simulink model "IEEE34_SPSload"  (R2021b)
settings: Solver=ode4  StartTime=0.0  StopTime=5  FixedStep=50e-6  RelTol=1e-3
PreLoadFcn:
  | pGain = 0.05; % Gain of random perturbation (pu)
  | pGainAP = 0.01; % Gain of sinusoidal active power variation (pu)
  | pGainRP = 0.01; % Gain of sinusoidal reactive power variation (pu)
  | pFreqAP = 0.03; % Frequency of sinusoidal active power variation (Hz)
  | pFreqRP = 0.03; % Frequency of sinusoidal reactive power variation (Hz)
  | 
  | init_IEEE34nodetestfeeder;
InitFcn:
  | pGain = 0.05; % Gain of random perturbation (pu)
  | pGainAP = 0.01; % Gain of sinusoidal active power variation (pu)
  | pGainRP = 0.01; % Gain of sinusoidal reactive power variation (pu)
  | pFreqAP = 0.03; % Frequency of sinusoidal active power variation (Hz)
  | pFreqRP = 0.03; % Frequency of sinusoidal reactive power variation (Hz)
  | 
  | init_IEEE34nodetestfeeder;
values from neighbouring files (symbols this model uses):
  fNom = f    (= 60)    [init_IEEE34nodetestfeeder.m]
  loadcoeff = 1.0    (= 1)    [init_IEEE34nodetestfeeder.m]
  Ts = 50e-6    (= 5e-05)    [init_IEEE34nodetestfeeder.m]
  vNomMV = VsubL    (= 24900)    [init_IEEE34nodetestfeeder.m]
  VsubL = 24.9e3    (= 24900)    [init_IEEE34nodetestfeeder.m]
  VxfmL = 4.16e3    (= 4160)    [init_IEEE34nodetestfeeder.m]
undefined symbols (not defined in the file or in its folder): Ac, Bc, Cc, Dc, find_system, j
libraries: spsSeriesRLCBranchLib x418, spsGroundLib x242, simulink_extras x176, spsVoltageMeasurementLib x106, spsRMSLib x96, spsControlledCurrentSourceLib x94, spsThreePhaseVIMeasurementLib x37, spsMutualInductanceLib x24, spsCurrentMeasurementLib x12, spsOnDelayLib x12, spsLinearTransformerLib x6, spsControlledVoltageSourceLib x6
(part 8 of 33)

== system IEEE34_SPSload/SM_IEEE34/Spot 830 ==
  Load B : Subsystem  DialogController=POWERSYS.PowerSysDialog  mask(Single-Phase Dynamic Load){NominalVoltage=[ VsubL 60 ], ActiveReactivePowers=[10*1000*loadcoeff 5*1000*loadcoeff], PositiveSequence=[1 0], ExternalControl=off, NpNq=[2 2], TimeConstants=[0  0  0  0], MinimumVoltage=0.7, LoadFlowParameters=[4,0,0,0,0]}
      mask prompts: NominalVoltage "Nominal voltage and frequency  [Vn(Vrms) fn(Hz)]:"; ActiveReactivePowers "Active and reactive power at initial voltage [Po(W) Qo(var)]:"; PositiveSequence "Initial voltage Vo [Mag(pu) Phase (deg.)]:"; ExternalControl "External control of PQ"; NpNq "Parameters [ np  nq ]:"; TimeConstants "Time constants [Tp1 Tp2 Tq1 Tq2]  (s):"; MinimumVoltage "Minimum voltage Vmin (pu):"; LoadFlowParameters "Load Flow parameters"
      mask help:
      | Implements a single-phase dynamic load. Active  power P and reactive
      | power Q absorbed by the load vary as function of voltage V  according to the
      | following equations:
      |
      |   If V>Vmin, P and Q vary as follows:
      |        P = Po * (V/Vo)^np * (1+Tp1.s)/(1+Tp2.s)
      |        Q = Qo * (V/Vo)^nq * (1+Tq1.s)/(1+Tq2.s)
      |   if V<Vmin
      |      Same equations with np=nq=2 (constant impedance load)
      mask init: same as IEEE34_SPSload/SM_IEEE34/DL836-1/Load B
      mask Help: helpview(psbhelp)
      mask Callback ExternalControl: powericon('ThreePhaseDynamicLoadCback',gcb);
      mask Display:
      | plot(-45,-45,45,45,[0,9,18,24,29,30,29,24,18,9,0,-9,-18,-24,-29,-30,-29,-24,-18,-9,0]*.9,[30,29,24,18,9,0,-9,-18,-24,-29,-30,-29,-24,-18,-9,0,9,18,24,29,30]*.9)
      | plot([0,0,10,0,-10,0]*1.1,[15,-5,-5,-15,-5,-5]*1.1)
  Load B1 : Subsystem  DialogController=POWERSYS.PowerSysDialog  mask(Single-Phase Dynamic Load){NominalVoltage=[ VsubL 60 ], ActiveReactivePowers=[10*1000*loadcoeff 5*1000*loadcoeff], PositiveSequence=[1 0], ExternalControl=off, NpNq=[2 2], TimeConstants=[0  0  0  0], MinimumVoltage=0.7, LoadFlowParameters=[4,0,0,0,0]}
      mask prompts: NominalVoltage "Nominal voltage and frequency  [Vn(Vrms) fn(Hz)]:"; ActiveReactivePowers "Active and reactive power at initial voltage [Po(W) Qo(var)]:"; PositiveSequence "Initial voltage Vo [Mag(pu) Phase (deg.)]:"; ExternalControl "External control of PQ"; NpNq "Parameters [ np  nq ]:"; TimeConstants "Time constants [Tp1 Tp2 Tq1 Tq2]  (s):"; MinimumVoltage "Minimum voltage Vmin (pu):"; LoadFlowParameters "Load Flow parameters"
      mask help:
      | Implements a single-phase dynamic load. Active  power P and reactive
      | power Q absorbed by the load vary as function of voltage V  according to the
      | following equations:
      |
      |   If V>Vmin, P and Q vary as follows:
      |        P = Po * (V/Vo)^np * (1+Tp1.s)/(1+Tp2.s)
      |        Q = Qo * (V/Vo)^nq * (1+Tq1.s)/(1+Tq2.s)
      |   if V<Vmin
      |      Same equations with np=nq=2 (constant impedance load)
      mask init: same as IEEE34_SPSload/SM_IEEE34/DL836-1/Load B
      mask Help: helpview(psbhelp)
      mask Callback ExternalControl: powericon('ThreePhaseDynamicLoadCback',gcb);
      mask Display:
      | plot(-45,-45,45,45,[0,9,18,24,29,30,29,24,18,9,0,-9,-18,-24,-29,-30,-29,-24,-18,-9,0]*.9,[30,29,24,18,9,0,-9,-18,-24,-29,-30,-29,-24,-18,-9,0,9,18,24,29,30]*.9)
      | plot([0,0,10,0,-10,0]*1.1,[15,-5,-5,-15,-5,-5]*1.1)
  Load B2 : Subsystem  DialogController=POWERSYS.PowerSysDialog  mask(Single-Phase Dynamic Load){NominalVoltage=[ VsubL 60 ], ActiveReactivePowers=[25*1000*loadcoeff 10*1000*loadcoeff], PositiveSequence=[1 0], ExternalControl=off, NpNq=[2 2], TimeConstants=[0  0  0  0], MinimumVoltage=0.7, LoadFlowParameters=[4,0,0,0,0]}
      mask prompts: NominalVoltage "Nominal voltage and frequency  [Vn(Vrms) fn(Hz)]:"; ActiveReactivePowers "Active and reactive power at initial voltage [Po(W) Qo(var)]:"; PositiveSequence "Initial voltage Vo [Mag(pu) Phase (deg.)]:"; ExternalControl "External control of PQ"; NpNq "Parameters [ np  nq ]:"; TimeConstants "Time constants [Tp1 Tp2 Tq1 Tq2]  (s):"; MinimumVoltage "Minimum voltage Vmin (pu):"; LoadFlowParameters "Load Flow parameters"
      mask help:
      | Implements a single-phase dynamic load. Active  power P and reactive
      | power Q absorbed by the load vary as function of voltage V  according to the
      | following equations:
      |
      |   If V>Vmin, P and Q vary as follows:
      |        P = Po * (V/Vo)^np * (1+Tp1.s)/(1+Tp2.s)
      |        Q = Qo * (V/Vo)^nq * (1+Tq1.s)/(1+Tq2.s)
      |   if V<Vmin
      |      Same equations with np=nq=2 (constant impedance load)
      mask init: same as IEEE34_SPSload/SM_IEEE34/DL836-1/Load B
      mask Help: helpview(psbhelp)
      mask Callback ExternalControl: powericon('ThreePhaseDynamicLoadCback',gcb);
      mask Display:
      | plot(-45,-45,45,45,[0,9,18,24,29,30,29,24,18,9,0,-9,-18,-24,-29,-30,-29,-24,-18,-9,0]*.9,[30,29,24,18,9,0,-9,-18,-24,-29,-30,-29,-24,-18,-9,0,9,18,24,29,30]*.9)
      | plot([0,0,10,0,-10,0]*1.1,[15,-5,-5,-15,-5,-5]*1.1)
  Terminator : Terminator
  Terminator1 : Terminator
  Terminator2 : Terminator
  A : PMIOPort  Side=Right
  B : PMIOPort  Port=2  Side=Right
  C : PMIOPort  Port=3  Side=Right
  wires:
  Load B/1(m) -> Terminator/1
  Load B1/1(m) -> Terminator1/1
  Load B2/1(m) -> Terminator2/1
  connections:
  A/RConn1 -- Load B2/LConn2 -- Load B/LConn1
  B/RConn1 -- Load B/LConn2 -- Load B1/LConn1
  C/RConn1 -- Load B1/LConn2 -- Load B2/LConn1

== system IEEE34_SPSload/SM_IEEE34/Spot 840 ==
  Ground4 : spsGroundLib/Ground  LConnTagsString=a
  Ground5 : spsGroundLib/Ground  LConnTagsString=a
  Ground6 : spsGroundLib/Ground  LConnTagsString=a
  Load B : Subsystem  DialogController=POWERSYS.PowerSysDialog  mask(Single-Phase Dynamic Load){NominalVoltage=[ VsubL/sqrt(3) 60 ], ActiveReactivePowers=[9*1000*loadcoeff 7*1000*loadcoeff], PositiveSequence=[1 0], ExternalControl=off, NpNq=[1 1], TimeConstants=[0  0  0  0], MinimumVoltage=0.7, LoadFlowParameters=[4,0,0,0,0]}
      mask prompts: NominalVoltage "Nominal voltage and frequency  [Vn(Vrms) fn(Hz)]:"; ActiveReactivePowers "Active and reactive power at initial voltage [Po(W) Qo(var)]:"; PositiveSequence "Initial voltage Vo [Mag(pu) Phase (deg.)]:"; ExternalControl "External control of PQ"; NpNq "Parameters [ np  nq ]:"; TimeConstants "Time constants [Tp1 Tp2 Tq1 Tq2]  (s):"; MinimumVoltage "Minimum voltage Vmin (pu):"; LoadFlowParameters "Load Flow parameters"
      mask help:
      | Implements a single-phase dynamic load. Active  power P and reactive
      | power Q absorbed by the load vary as function of voltage V  according to the
      | following equations:
      |
      |   If V>Vmin, P and Q vary as follows:
      |        P = Po * (V/Vo)^np * (1+Tp1.s)/(1+Tp2.s)
      |        Q = Qo * (V/Vo)^nq * (1+Tq1.s)/(1+Tq2.s)
      |   if V<Vmin
      |      Same equations with np=nq=2 (constant impedance load)
      mask init: same as IEEE34_SPSload/SM_IEEE34/DL836-1/Load B
      mask Help: helpview(psbhelp)
      mask Callback ExternalControl: powericon('ThreePhaseDynamicLoadCback',gcb);
      mask Display:
      | plot(-45,-45,45,45,[0,9,18,24,29,30,29,24,18,9,0,-9,-18,-24,-29,-30,-29,-24,-18,-9,0]*.9,[30,29,24,18,9,0,-9,-18,-24,-29,-30,-29,-24,-18,-9,0,9,18,24,29,30]*.9)
      | plot([0,0,10,0,-10,0]*1.1,[15,-5,-5,-15,-5,-5]*1.1)
  Load B1 : Subsystem  DialogController=POWERSYS.PowerSysDialog  mask(Single-Phase Dynamic Load){NominalVoltage=[ VsubL/sqrt(3) 60 ], ActiveReactivePowers=[9*1000*loadcoeff 7*1000*loadcoeff], PositiveSequence=[1 0], ExternalControl=off, NpNq=[1 1], TimeConstants=[0  0  0  0], MinimumVoltage=0.7, LoadFlowParameters=[4,0,0,0,0]}
      mask prompts: NominalVoltage "Nominal voltage and frequency  [Vn(Vrms) fn(Hz)]:"; ActiveReactivePowers "Active and reactive power at initial voltage [Po(W) Qo(var)]:"; PositiveSequence "Initial voltage Vo [Mag(pu) Phase (deg.)]:"; ExternalControl "External control of PQ"; NpNq "Parameters [ np  nq ]:"; TimeConstants "Time constants [Tp1 Tp2 Tq1 Tq2]  (s):"; MinimumVoltage "Minimum voltage Vmin (pu):"; LoadFlowParameters "Load Flow parameters"
      mask help:
      | Implements a single-phase dynamic load. Active  power P and reactive
      | power Q absorbed by the load vary as function of voltage V  according to the
      | following equations:
      |
      |   If V>Vmin, P and Q vary as follows:
      |        P = Po * (V/Vo)^np * (1+Tp1.s)/(1+Tp2.s)
      |        Q = Qo * (V/Vo)^nq * (1+Tq1.s)/(1+Tq2.s)
      |   if V<Vmin
      |      Same equations with np=nq=2 (constant impedance load)
      mask init: same as IEEE34_SPSload/SM_IEEE34/DL836-1/Load B
      mask Help: helpview(psbhelp)
      mask Callback ExternalControl: powericon('ThreePhaseDynamicLoadCback',gcb);
      mask Display:
      | plot(-45,-45,45,45,[0,9,18,24,29,30,29,24,18,9,0,-9,-18,-24,-29,-30,-29,-24,-18,-9,0]*.9,[30,29,24,18,9,0,-9,-18,-24,-29,-30,-29,-24,-18,-9,0,9,18,24,29,30]*.9)
      | plot([0,0,10,0,-10,0]*1.1,[15,-5,-5,-15,-5,-5]*1.1)
  Load B2 : Subsystem  DialogController=POWERSYS.PowerSysDialog  mask(Single-Phase Dynamic Load){NominalVoltage=[ VsubL/sqrt(3) 60 ], ActiveReactivePowers=[9*1000*loadcoeff 7*1000*loadcoeff], PositiveSequence=[1 0], ExternalControl=off, NpNq=[1 1], TimeConstants=[0  0  0  0], MinimumVoltage=0.7, LoadFlowParameters=[4,0,0,0,0]}
      mask prompts: NominalVoltage "Nominal voltage and frequency  [Vn(Vrms) fn(Hz)]:"; ActiveReactivePowers "Active and reactive power at initial voltage [Po(W) Qo(var)]:"; PositiveSequence "Initial voltage Vo [Mag(pu) Phase (deg.)]:"; ExternalControl "External control of PQ"; NpNq "Parameters [ np  nq ]:"; TimeConstants "Time constants [Tp1 Tp2 Tq1 Tq2]  (s):"; MinimumVoltage "Minimum voltage Vmin (pu):"; LoadFlowParameters "Load Flow parameters"
      mask help:
      | Implements a single-phase dynamic load. Active  power P and reactive
      | power Q absorbed by the load vary as function of voltage V  according to the
      | following equations:
      |
      |   If V>Vmin, P and Q vary as follows:
      |        P = Po * (V/Vo)^np * (1+Tp1.s)/(1+Tp2.s)
      |        Q = Qo * (V/Vo)^nq * (1+Tq1.s)/(1+Tq2.s)
      |   if V<Vmin
      |      Same equations with np=nq=2 (constant impedance load)
      mask init: same as IEEE34_SPSload/SM_IEEE34/DL836-1/Load B
      mask Help: helpview(psbhelp)
      mask Callback ExternalControl: powericon('ThreePhaseDynamicLoadCback',gcb);
      mask Display:
      | plot(-45,-45,45,45,[0,9,18,24,29,30,29,24,18,9,0,-9,-18,-24,-29,-30,-29,-24,-18,-9,0]*.9,[30,29,24,18,9,0,-9,-18,-24,-29,-30,-29,-24,-18,-9,0,9,18,24,29,30]*.9)
      | plot([0,0,10,0,-10,0]*1.1,[15,-5,-5,-15,-5,-5]*1.1)
  Terminator : Terminator
  Terminator1 : Terminator
  Terminator2 : Terminator
  A : PMIOPort  Side=Right
  B : PMIOPort  Port=2  Side=Right
  C : PMIOPort  Port=3  Side=Right
  wires:
  Load B/1(m) -> Terminator/1
  Load B1/1(m) -> Terminator1/1
  Load B2/1(m) -> Terminator2/1
  connections:
  Load B/LConn2 -- Ground4/LConn1
  A/RConn1 -- Load B/LConn1
  Load B1/LConn2 -- Ground5/LConn1
  B/RConn1 -- Load B1/LConn1
  C/RConn1 -- Load B2/LConn1
  Load B2/LConn2 -- Ground6/LConn1

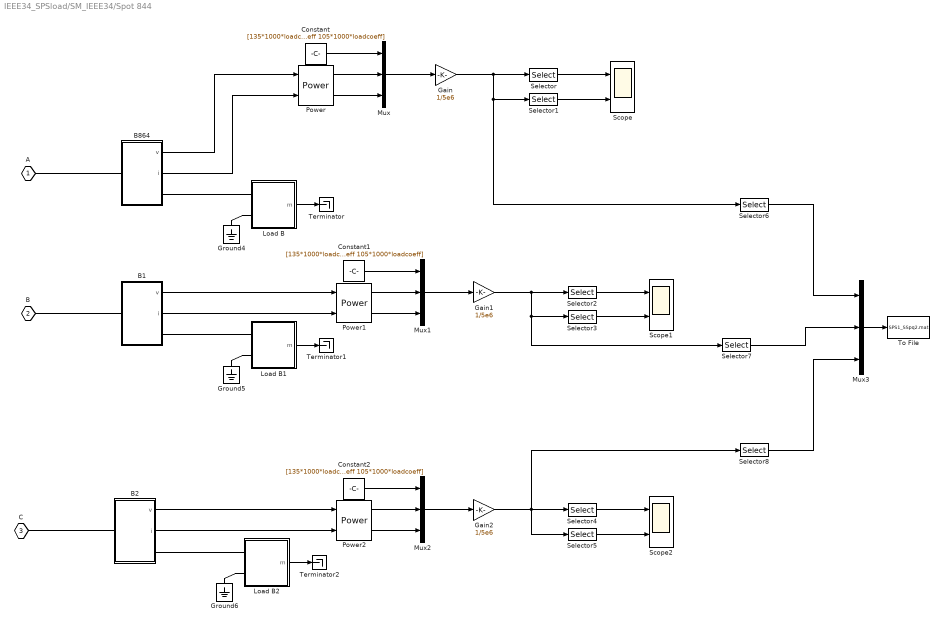
== system IEEE34_SPSload/SM_IEEE34/Spot 844 ==
  B1 : Subsystem
  B2 : Subsystem
  B864 : Subsystem
  Constant : Constant  Value=[135*1000*loadcoeff 105*1000*loadcoeff]
  Constant1 : Constant  Value=[135*1000*loadcoeff 105*1000*loadcoeff]
  Constant2 : Constant  Value=[135*1000*loadcoeff 105*1000*loadcoeff]
  Gain : Gain  Gain=1/5e6
  Gain1 : Gain  Gain=1/5e6
  Gain2 : Gain  Gain=1/5e6
  Ground4 : spsGroundLib/Ground  LConnTagsString=a
  Ground5 : spsGroundLib/Ground  LConnTagsString=a
  Ground6 : spsGroundLib/Ground  LConnTagsString=a
  Load B : Subsystem  DialogController=POWERSYS.PowerSysDialog  mask(Single-Phase Dynamic Load){NominalVoltage=[ VsubL/sqrt(3) 60 ], ActiveReactivePowers=[135*1000*loadcoeff 105*1000*loadcoeff], PositiveSequence=[1 0], ExternalControl=off, NpNq=[2 2], TimeConstants=[0  0  0  0], MinimumVoltage=0.7, LoadFlowParameters=[4,0,0,0,0]}
      mask prompts: NominalVoltage "Nominal voltage and frequency  [Vn(Vrms) fn(Hz)]:"; ActiveReactivePowers "Active and reactive power at initial voltage [Po(W) Qo(var)]:"; PositiveSequence "Initial voltage Vo [Mag(pu) Phase (deg.)]:"; ExternalControl "External control of PQ"; NpNq "Parameters [ np  nq ]:"; TimeConstants "Time constants [Tp1 Tp2 Tq1 Tq2]  (s):"; MinimumVoltage "Minimum voltage Vmin (pu):"; LoadFlowParameters "Load Flow parameters"
      mask help:
      | Implements a single-phase dynamic load. Active  power P and reactive
      | power Q absorbed by the load vary as function of voltage V  according to the
      | following equations:
      |
      |   If V>Vmin, P and Q vary as follows:
      |        P = Po * (V/Vo)^np * (1+Tp1.s)/(1+Tp2.s)
      |        Q = Qo * (V/Vo)^nq * (1+Tq1.s)/(1+Tq2.s)
      |   if V<Vmin
      |      Same equations with np=nq=2 (constant impedance load)
      mask init: same as IEEE34_SPSload/SM_IEEE34/DL836-1/Load B
      mask Help: helpview(psbhelp)
      mask Callback ExternalControl: powericon('ThreePhaseDynamicLoadCback',gcb);
      mask Display:
      | plot(-45,-45,45,45,[0,9,18,24,29,30,29,24,18,9,0,-9,-18,-24,-29,-30,-29,-24,-18,-9,0]*.9,[30,29,24,18,9,0,-9,-18,-24,-29,-30,-29,-24,-18,-9,0,9,18,24,29,30]*.9)
      | plot([0,0,10,0,-10,0]*1.1,[15,-5,-5,-15,-5,-5]*1.1)
  Load B1 : Subsystem  DialogController=POWERSYS.PowerSysDialog  mask(Single-Phase Dynamic Load){NominalVoltage=[ VsubL/sqrt(3) 60 ], ActiveReactivePowers=[135*1000*loadcoeff 105*1000*loadcoeff], PositiveSequence=[1 0], ExternalControl=off, NpNq=[2 2], TimeConstants=[0  0  0  0], MinimumVoltage=0.7, LoadFlowParameters=[4,0,0,0,0]}
      mask prompts: NominalVoltage "Nominal voltage and frequency  [Vn(Vrms) fn(Hz)]:"; ActiveReactivePowers "Active and reactive power at initial voltage [Po(W) Qo(var)]:"; PositiveSequence "Initial voltage Vo [Mag(pu) Phase (deg.)]:"; ExternalControl "External control of PQ"; NpNq "Parameters [ np  nq ]:"; TimeConstants "Time constants [Tp1 Tp2 Tq1 Tq2]  (s):"; MinimumVoltage "Minimum voltage Vmin (pu):"; LoadFlowParameters "Load Flow parameters"
      mask help:
      | Implements a single-phase dynamic load. Active  power P and reactive
      | power Q absorbed by the load vary as function of voltage V  according to the
      | following equations:
      |
      |   If V>Vmin, P and Q vary as follows:
      |        P = Po * (V/Vo)^np * (1+Tp1.s)/(1+Tp2.s)
      |        Q = Qo * (V/Vo)^nq * (1+Tq1.s)/(1+Tq2.s)
      |   if V<Vmin
      |      Same equations with np=nq=2 (constant impedance load)
      mask init: same as IEEE34_SPSload/SM_IEEE34/DL836-1/Load B
      mask Help: helpview(psbhelp)
      mask Callback ExternalControl: powericon('ThreePhaseDynamicLoadCback',gcb);
      mask Display:
      | plot(-45,-45,45,45,[0,9,18,24,29,30,29,24,18,9,0,-9,-18,-24,-29,-30,-29,-24,-18,-9,0]*.9,[30,29,24,18,9,0,-9,-18,-24,-29,-30,-29,-24,-18,-9,0,9,18,24,29,30]*.9)
      | plot([0,0,10,0,-10,0]*1.1,[15,-5,-5,-15,-5,-5]*1.1)
  Load B2 : Subsystem  DialogController=POWERSYS.PowerSysDialog  mask(Single-Phase Dynamic Load){NominalVoltage=[ VsubL/sqrt(3) 60 ], ActiveReactivePowers=[135*1000*loadcoeff 105*1000*loadcoeff], PositiveSequence=[1 0], ExternalControl=off, NpNq=[2 2], TimeConstants=[0  0  0  0], MinimumVoltage=0.7, LoadFlowParameters=[4,0,0,0,0]}
      mask prompts: NominalVoltage "Nominal voltage and frequency  [Vn(Vrms) fn(Hz)]:"; ActiveReactivePowers "Active and reactive power at initial voltage [Po(W) Qo(var)]:"; PositiveSequence "Initial voltage Vo [Mag(pu) Phase (deg.)]:"; ExternalControl "External control of PQ"; NpNq "Parameters [ np  nq ]:"; TimeConstants "Time constants [Tp1 Tp2 Tq1 Tq2]  (s):"; MinimumVoltage "Minimum voltage Vmin (pu):"; LoadFlowParameters "Load Flow parameters"
      mask help:
      | Implements a single-phase dynamic load. Active  power P and reactive
      | power Q absorbed by the load vary as function of voltage V  according to the
      | following equations:
      |
      |   If V>Vmin, P and Q vary as follows:
      |        P = Po * (V/Vo)^np * (1+Tp1.s)/(1+Tp2.s)
      |        Q = Qo * (V/Vo)^nq * (1+Tq1.s)/(1+Tq2.s)
      |   if V<Vmin
      |      Same equations with np=nq=2 (constant impedance load)
      mask init: same as IEEE34_SPSload/SM_IEEE34/DL836-1/Load B
      mask Help: helpview(psbhelp)
      mask Callback ExternalControl: powericon('ThreePhaseDynamicLoadCback',gcb);
      mask Display:
      | plot(-45,-45,45,45,[0,9,18,24,29,30,29,24,18,9,0,-9,-18,-24,-29,-30,-29,-24,-18,-9,0]*.9,[30,29,24,18,9,0,-9,-18,-24,-29,-30,-29,-24,-18,-9,0,9,18,24,29,30]*.9)
      | plot([0,0,10,0,-10,0]*1.1,[15,-5,-5,-15,-5,-5]*1.1)
  Mux{,1..3} (4 alike) : Mux  Inputs=3
  Power : spsPowerLib/Power  Freq=60  Vinit=[1, 0]  Iinit=[1, 0]  Ts=0
      settings: SourceProductBaseCode=PS
  Power1 : spsPowerLib/Power  Freq=60  Vinit=[1, 0]  Iinit=[1, 0]  Ts=0
      settings: SourceProductBaseCode=PS
  Power2 : spsPowerLib/Power  Freq=60  Vinit=[1, 0]  Iinit=[1, 0]  Ts=0
      settings: SourceProductBaseCode=PS
  Scope : Scope  NumInputPorts=2
  Scope1 : Scope  NumInputPorts=2
  Scope2 : Scope  NumInputPorts=2
  Selector : Selector  InputPortWidth=4  IndexOptions=Index vector (dialog)  Indices=[1 3]  OutputSizes=1
  Selector1 : Selector  InputPortWidth=4  IndexOptions=Index vector (dialog)  Indices=[2 4]  OutputSizes=1
  Selector2 : Selector  InputPortWidth=4  IndexOptions=Index vector (dialog)  Indices=[1 3]  OutputSizes=1
  Selector3 : Selector  InputPortWidth=4  IndexOptions=Index vector (dialog)  Indices=[2 4]  OutputSizes=1
  Selector4 : Selector  InputPortWidth=4  IndexOptions=Index vector (dialog)  Indices=[1 3]  OutputSizes=1
  Selector5 : Selector  InputPortWidth=4  IndexOptions=Index vector (dialog)  Indices=[2 4]  OutputSizes=1
  Selector6 : Selector  InputPortWidth=4  IndexOptions=Index vector (dialog)  Indices=[3 4]  OutputSizes=1
  Selector7 : Selector  InputPortWidth=4  IndexOptions=Index vector (dialog)  Indices=[3 4]  OutputSizes=1
  Selector8 : Selector  InputPortWidth=4  IndexOptions=Index vector (dialog)  Indices=[3 4]  OutputSizes=1
  Terminator : Terminator
  Terminator1 : Terminator
  Terminator2 : Terminator
  To File : ToFile  Filename=SPS1_SSpq2.mat  MatrixName=SPS1_SSpq2
  A : PMIOPort  Side=Right
  B : PMIOPort  Port=2  Side=Right
  C : PMIOPort  Port=3  Side=Right
  wires:
  Load B/1(m) -> Terminator/1
  Load B1/1(m) -> Terminator1/1
  Load B2/1(m) -> Terminator2/1
  Gain/1 -> Selector6/1, Selector1/1, Selector/1
  B864/1(v) -> Power/1
  Mux/1 -> Gain/1
  Power/1 -> Mux/2
  B864/2(i) -> Power/2
  Selector/1 -> Scope/1
  Power/2 -> Mux/3
  Selector1/1 -> Scope/2
  Constant/1 -> Mux/1
  Constant1/1 -> Mux1/1
  Selector3/1 -> Scope1/2
  Power1/2 -> Mux1/3
  Selector2/1 -> Scope1/1
  Power1/1 -> Mux1/2
  Mux1/1 -> Gain1/1
  Gain1/1 -> Selector2/1, Selector7/1, Selector3/1
  Gain2/1 -> Selector8/1, Selector5/1, Selector4/1
  Mux2/1 -> Gain2/1
  Power2/1 -> Mux2/2
  Selector4/1 -> Scope2/1
  Power2/2 -> Mux2/3
  Selector5/1 -> Scope2/2
  Constant2/1 -> Mux2/1
  B2/1(v) -> Power2/1
  B2/2(i) -> Power2/2
  B1/1(v) -> Power1/1
  B1/2(i) -> Power1/2
  Mux3/1 -> To File/1
  Selector7/1 -> Mux3/2
  Selector8/1 -> Mux3/3
  Selector6/1 -> Mux3/1
  connections:
  Load B/LConn2 -- Ground4/LConn1
  Load B1/LConn2 -- Ground5/LConn1
  Load B2/LConn2 -- Ground6/LConn1
  B864/LConn1 -- A/RConn1
  B864/RConn1 -- Load B/LConn1
  B1/RConn1 -- Load B1/LConn1
  B2/RConn1 -- Load B2/LConn1
  B/RConn1 -- B1/LConn1
  C/RConn1 -- B2/LConn1

== system IEEE34_SPSload/SM_IEEE34/Spot 848 ==
  Load B : Subsystem  DialogController=POWERSYS.PowerSysDialog  mask(Single-Phase Dynamic Load){NominalVoltage=[ VsubL 60 ], ActiveReactivePowers=[20*1000*loadcoeff 16*1000*loadcoeff], PositiveSequence=[1 0], ExternalControl=off, NpNq=[0 0], TimeConstants=[0  0  0  0], MinimumVoltage=0.7, LoadFlowParameters=[4,0,0,0,0]}
      mask prompts: NominalVoltage "Nominal voltage and frequency  [Vn(Vrms) fn(Hz)]:"; ActiveReactivePowers "Active and reactive power at initial voltage [Po(W) Qo(var)]:"; PositiveSequence "Initial voltage Vo [Mag(pu) Phase (deg.)]:"; ExternalControl "External control of PQ"; NpNq "Parameters [ np  nq ]:"; TimeConstants "Time constants [Tp1 Tp2 Tq1 Tq2]  (s):"; MinimumVoltage "Minimum voltage Vmin (pu):"; LoadFlowParameters "Load Flow parameters"
      mask help:
      | Implements a single-phase dynamic load. Active  power P and reactive
      | power Q absorbed by the load vary as function of voltage V  according to the
      | following equations:
      |
      |   If V>Vmin, P and Q vary as follows:
      |        P = Po * (V/Vo)^np * (1+Tp1.s)/(1+Tp2.s)
      |        Q = Qo * (V/Vo)^nq * (1+Tq1.s)/(1+Tq2.s)
      |   if V<Vmin
      |      Same equations with np=nq=2 (constant impedance load)
      mask init: same as IEEE34_SPSload/SM_IEEE34/DL836-1/Load B
      mask Help: helpview(psbhelp)
      mask Callback ExternalControl: powericon('ThreePhaseDynamicLoadCback',gcb);
      mask Display:
      | plot(-45,-45,45,45,[0,9,18,24,29,30,29,24,18,9,0,-9,-18,-24,-29,-30,-29,-24,-18,-9,0]*.9,[30,29,24,18,9,0,-9,-18,-24,-29,-30,-29,-24,-18,-9,0,9,18,24,29,30]*.9)
      | plot([0,0,10,0,-10,0]*1.1,[15,-5,-5,-15,-5,-5]*1.1)
  Load B1 : Subsystem  DialogController=POWERSYS.PowerSysDialog  mask(Single-Phase Dynamic Load){NominalVoltage=[ VsubL 60 ], ActiveReactivePowers=[20*1000*loadcoeff 16*1000*loadcoeff], PositiveSequence=[1 0], ExternalControl=off, NpNq=[0 0], TimeConstants=[0  0  0  0], MinimumVoltage=0.7, LoadFlowParameters=[4,0,0,0,0]}
      mask prompts: NominalVoltage "Nominal voltage and frequency  [Vn(Vrms) fn(Hz)]:"; ActiveReactivePowers "Active and reactive power at initial voltage [Po(W) Qo(var)]:"; PositiveSequence "Initial voltage Vo [Mag(pu) Phase (deg.)]:"; ExternalControl "External control of PQ"; NpNq "Parameters [ np  nq ]:"; TimeConstants "Time constants [Tp1 Tp2 Tq1 Tq2]  (s):"; MinimumVoltage "Minimum voltage Vmin (pu):"; LoadFlowParameters "Load Flow parameters"
      mask help:
      | Implements a single-phase dynamic load. Active  power P and reactive
      | power Q absorbed by the load vary as function of voltage V  according to the
      | following equations:
      |
      |   If V>Vmin, P and Q vary as follows:
      |        P = Po * (V/Vo)^np * (1+Tp1.s)/(1+Tp2.s)
      |        Q = Qo * (V/Vo)^nq * (1+Tq1.s)/(1+Tq2.s)
      |   if V<Vmin
      |      Same equations with np=nq=2 (constant impedance load)
      mask init: same as IEEE34_SPSload/SM_IEEE34/DL836-1/Load B
      mask Help: helpview(psbhelp)
      mask Callback ExternalControl: powericon('ThreePhaseDynamicLoadCback',gcb);
      mask Display:
      | plot(-45,-45,45,45,[0,9,18,24,29,30,29,24,18,9,0,-9,-18,-24,-29,-30,-29,-24,-18,-9,0]*.9,[30,29,24,18,9,0,-9,-18,-24,-29,-30,-29,-24,-18,-9,0,9,18,24,29,30]*.9)
      | plot([0,0,10,0,-10,0]*1.1,[15,-5,-5,-15,-5,-5]*1.1)
  Load B2 : Subsystem  DialogController=POWERSYS.PowerSysDialog  mask(Single-Phase Dynamic Load){NominalVoltage=[ VsubL 60 ], ActiveReactivePowers=[20*1000*loadcoeff 16*1000*loadcoeff], PositiveSequence=[1 0], ExternalControl=off, NpNq=[0 0], TimeConstants=[0  0  0  0], MinimumVoltage=0.7, LoadFlowParameters=[4,0,0,0,0]}
      mask prompts: NominalVoltage "Nominal voltage and frequency  [Vn(Vrms) fn(Hz)]:"; ActiveReactivePowers "Active and reactive power at initial voltage [Po(W) Qo(var)]:"; PositiveSequence "Initial voltage Vo [Mag(pu) Phase (deg.)]:"; ExternalControl "External control of PQ"; NpNq "Parameters [ np  nq ]:"; TimeConstants "Time constants [Tp1 Tp2 Tq1 Tq2]  (s):"; MinimumVoltage "Minimum voltage Vmin (pu):"; LoadFlowParameters "Load Flow parameters"
      mask help:
      | Implements a single-phase dynamic load. Active  power P and reactive
      | power Q absorbed by the load vary as function of voltage V  according to the
      | following equations:
      |
      |   If V>Vmin, P and Q vary as follows:
      |        P = Po * (V/Vo)^np * (1+Tp1.s)/(1+Tp2.s)
      |        Q = Qo * (V/Vo)^nq * (1+Tq1.s)/(1+Tq2.s)
      |   if V<Vmin
      |      Same equations with np=nq=2 (constant impedance load)
      mask init: same as IEEE34_SPSload/SM_IEEE34/DL836-1/Load B
      mask Help: helpview(psbhelp)
      mask Callback ExternalControl: powericon('ThreePhaseDynamicLoadCback',gcb);
      mask Display:
      | plot(-45,-45,45,45,[0,9,18,24,29,30,29,24,18,9,0,-9,-18,-24,-29,-30,-29,-24,-18,-9,0]*.9,[30,29,24,18,9,0,-9,-18,-24,-29,-30,-29,-24,-18,-9,0,9,18,24,29,30]*.9)
      | plot([0,0,10,0,-10,0]*1.1,[15,-5,-5,-15,-5,-5]*1.1)
  Terminator : Terminator
  Terminator1 : Terminator
  Terminator2 : Terminator
  A : PMIOPort  Side=Right
  B : PMIOPort  Port=2  Side=Right
  C : PMIOPort  Port=3  Side=Right
  wires:
  Load B/1(m) -> Terminator/1
  Load B1/1(m) -> Terminator1/1
  Load B2/1(m) -> Terminator2/1
  connections:
  A/RConn1 -- Load B2/LConn2 -- Load B/LConn1
  B/RConn1 -- Load B/LConn2 -- Load B1/LConn1
  Load B2/LConn1 -- Load B1/LConn2 -- C/RConn1

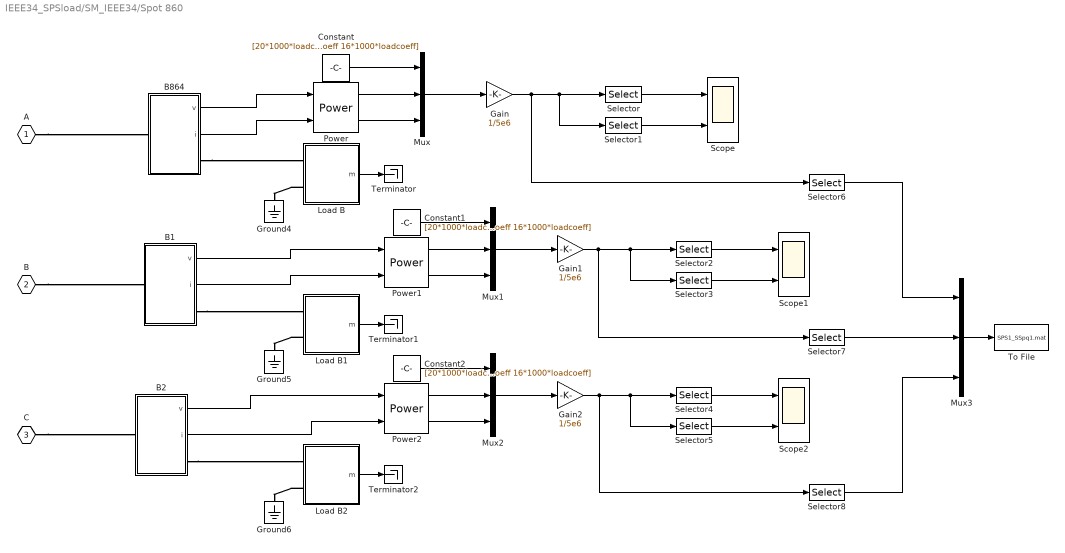
== system IEEE34_SPSload/SM_IEEE34/Spot 860 ==
  B1 : Subsystem
  B2 : Subsystem
  B864 : Subsystem
  Constant : Constant  Value=[20*1000*loadcoeff 16*1000*loadcoeff]
  Constant1 : Constant  Value=[20*1000*loadcoeff 16*1000*loadcoeff]
  Constant2 : Constant  Value=[20*1000*loadcoeff 16*1000*loadcoeff]
  Gain : Gain  Gain=1/5e6
  Gain1 : Gain  Gain=1/5e6
  Gain2 : Gain  Gain=1/5e6
  Ground4 : spsGroundLib/Ground  LConnTagsString=a
  Ground5 : spsGroundLib/Ground  LConnTagsString=a
  Ground6 : spsGroundLib/Ground  LConnTagsString=a
  Load B : Subsystem  DialogController=POWERSYS.PowerSysDialog  mask(Single-Phase Dynamic Load){NominalVoltage=[ VsubL/sqrt(3) 60 ], ActiveReactivePowers=[20*1000*loadcoeff 16*1000*loadcoeff], PositiveSequence=[1 0], ExternalControl=off, NpNq=[0 0], TimeConstants=[0  0  0  0], MinimumVoltage=0.7, LoadFlowParameters=[4,0,0,0,0]}
      mask prompts: NominalVoltage "Nominal voltage and frequency  [Vn(Vrms) fn(Hz)]:"; ActiveReactivePowers "Active and reactive power at initial voltage [Po(W) Qo(var)]:"; PositiveSequence "Initial voltage Vo [Mag(pu) Phase (deg.)]:"; ExternalControl "External control of PQ"; NpNq "Parameters [ np  nq ]:"; TimeConstants "Time constants [Tp1 Tp2 Tq1 Tq2]  (s):"; MinimumVoltage "Minimum voltage Vmin (pu):"; LoadFlowParameters "Load Flow parameters"
      mask help:
      | Implements a single-phase dynamic load. Active  power P and reactive
      | power Q absorbed by the load vary as function of voltage V  according to the
      | following equations:
      |
      |   If V>Vmin, P and Q vary as follows:
      |        P = Po * (V/Vo)^np * (1+Tp1.s)/(1+Tp2.s)
      |        Q = Qo * (V/Vo)^nq * (1+Tq1.s)/(1+Tq2.s)
      |   if V<Vmin
      |      Same equations with np=nq=2 (constant impedance load)
      mask init: same as IEEE34_SPSload/SM_IEEE34/DL836-1/Load B
      mask Help: helpview(psbhelp)
      mask Callback ExternalControl: powericon('ThreePhaseDynamicLoadCback',gcb);
      mask Display:
      | plot(-45,-45,45,45,[0,9,18,24,29,30,29,24,18,9,0,-9,-18,-24,-29,-30,-29,-24,-18,-9,0]*.9,[30,29,24,18,9,0,-9,-18,-24,-29,-30,-29,-24,-18,-9,0,9,18,24,29,30]*.9)
      | plot([0,0,10,0,-10,0]*1.1,[15,-5,-5,-15,-5,-5]*1.1)
  Load B1 : Subsystem  DialogController=POWERSYS.PowerSysDialog  mask(Single-Phase Dynamic Load){NominalVoltage=[ VsubL/sqrt(3) 60 ], ActiveReactivePowers=[20*1000*loadcoeff 16*1000*loadcoeff], PositiveSequence=[1 0], ExternalControl=off, NpNq=[0 0], TimeConstants=[0  0  0  0], MinimumVoltage=0.7, LoadFlowParameters=[4,0,0,0,0]}
      mask prompts: NominalVoltage "Nominal voltage and frequency  [Vn(Vrms) fn(Hz)]:"; ActiveReactivePowers "Active and reactive power at initial voltage [Po(W) Qo(var)]:"; PositiveSequence "Initial voltage Vo [Mag(pu) Phase (deg.)]:"; ExternalControl "External control of PQ"; NpNq "Parameters [ np  nq ]:"; TimeConstants "Time constants [Tp1 Tp2 Tq1 Tq2]  (s):"; MinimumVoltage "Minimum voltage Vmin (pu):"; LoadFlowParameters "Load Flow parameters"
      mask help:
      | Implements a single-phase dynamic load. Active  power P and reactive
      | power Q absorbed by the load vary as function of voltage V  according to the
      | following equations:
      |
      |   If V>Vmin, P and Q vary as follows:
      |        P = Po * (V/Vo)^np * (1+Tp1.s)/(1+Tp2.s)
      |        Q = Qo * (V/Vo)^nq * (1+Tq1.s)/(1+Tq2.s)
      |   if V<Vmin
      |      Same equations with np=nq=2 (constant impedance load)
      mask init: same as IEEE34_SPSload/SM_IEEE34/DL836-1/Load B
      mask Help: helpview(psbhelp)
      mask Callback ExternalControl: powericon('ThreePhaseDynamicLoadCback',gcb);
      mask Display:
      | plot(-45,-45,45,45,[0,9,18,24,29,30,29,24,18,9,0,-9,-18,-24,-29,-30,-29,-24,-18,-9,0]*.9,[30,29,24,18,9,0,-9,-18,-24,-29,-30,-29,-24,-18,-9,0,9,18,24,29,30]*.9)
      | plot([0,0,10,0,-10,0]*1.1,[15,-5,-5,-15,-5,-5]*1.1)
  Load B2 : Subsystem  DialogController=POWERSYS.PowerSysDialog  mask(Single-Phase Dynamic Load){NominalVoltage=[ VsubL/sqrt(3) 60 ], ActiveReactivePowers=[20*1000*loadcoeff 16*1000*loadcoeff], PositiveSequence=[1 0], ExternalControl=off, NpNq=[0 0], TimeConstants=[0  0  0  0], MinimumVoltage=0.7, LoadFlowParameters=[4,0,0,0,0]}
      mask prompts: NominalVoltage "Nominal voltage and frequency  [Vn(Vrms) fn(Hz)]:"; ActiveReactivePowers "Active and reactive power at initial voltage [Po(W) Qo(var)]:"; PositiveSequence "Initial voltage Vo [Mag(pu) Phase (deg.)]:"; ExternalControl "External control of PQ"; NpNq "Parameters [ np  nq ]:"; TimeConstants "Time constants [Tp1 Tp2 Tq1 Tq2]  (s):"; MinimumVoltage "Minimum voltage Vmin (pu):"; LoadFlowParameters "Load Flow parameters"
      mask help:
      | Implements a single-phase dynamic load. Active  power P and reactive
      | power Q absorbed by the load vary as function of voltage V  according to the
      | following equations:
      |
      |   If V>Vmin, P and Q vary as follows:
      |        P = Po * (V/Vo)^np * (1+Tp1.s)/(1+Tp2.s)
      |        Q = Qo * (V/Vo)^nq * (1+Tq1.s)/(1+Tq2.s)
      |   if V<Vmin
      |      Same equations with np=nq=2 (constant impedance load)
      mask init: same as IEEE34_SPSload/SM_IEEE34/DL836-1/Load B
      mask Help: helpview(psbhelp)
      mask Callback ExternalControl: powericon('ThreePhaseDynamicLoadCback',gcb);
      mask Display:
      | plot(-45,-45,45,45,[0,9,18,24,29,30,29,24,18,9,0,-9,-18,-24,-29,-30,-29,-24,-18,-9,0]*.9,[30,29,24,18,9,0,-9,-18,-24,-29,-30,-29,-24,-18,-9,0,9,18,24,29,30]*.9)
      | plot([0,0,10,0,-10,0]*1.1,[15,-5,-5,-15,-5,-5]*1.1)
  Mux{,1..3} (4 alike) : Mux  Inputs=3
  Power : spsPowerLib/Power  Freq=60  Vinit=[1, 0]  Iinit=[1, 0]  Ts=0
      settings: SourceProductBaseCode=PS
  Power1 : spsPowerLib/Power  Freq=60  Vinit=[1, 0]  Iinit=[1, 0]  Ts=0
      settings: SourceProductBaseCode=PS
  Power2 : spsPowerLib/Power  Freq=60  Vinit=[1, 0]  Iinit=[1, 0]  Ts=0
      settings: SourceProductBaseCode=PS
  Scope : Scope  NumInputPorts=2
  Scope1 : Scope  NumInputPorts=2
  Scope2 : Scope  NumInputPorts=2
  Selector : Selector  InputPortWidth=4  IndexOptions=Index vector (dialog)  Indices=[1 3]  OutputSizes=1
  Selector1 : Selector  InputPortWidth=4  IndexOptions=Index vector (dialog)  Indices=[2 4]  OutputSizes=1
  Selector2 : Selector  InputPortWidth=4  IndexOptions=Index vector (dialog)  Indices=[1 3]  OutputSizes=1
  Selector3 : Selector  InputPortWidth=4  IndexOptions=Index vector (dialog)  Indices=[2 4]  OutputSizes=1
  Selector4 : Selector  InputPortWidth=4  IndexOptions=Index vector (dialog)  Indices=[1 3]  OutputSizes=1
  Selector5 : Selector  InputPortWidth=4  IndexOptions=Index vector (dialog)  Indices=[2 4]  OutputSizes=1
  Selector6 : Selector  InputPortWidth=4  IndexOptions=Index vector (dialog)  Indices=[3 4]  OutputSizes=1
  Selector7 : Selector  InputPortWidth=4  IndexOptions=Index vector (dialog)  Indices=[3 4]  OutputSizes=1
  Selector8 : Selector  InputPortWidth=4  IndexOptions=Index vector (dialog)  Indices=[3 4]  OutputSizes=1
  Terminator : Terminator
  Terminator1 : Terminator
  Terminator2 : Terminator
  To File : ToFile  Filename=SPS1_SSpq1.mat  MatrixName=SPS1_SSpq1
  A : PMIOPort  Side=Right
  B : PMIOPort  Port=2  Side=Right
  C : PMIOPort  Port=3  Side=Right
  wires:
  Load B/1(m) -> Terminator/1
  Load B1/1(m) -> Terminator1/1
  Load B2/1(m) -> Terminator2/1
  Selector1/1 -> Scope/2
  Gain/1 -> Selector6/1, Selector1/1, Selector/1
  Selector/1 -> Scope/1
  Power/2 -> Mux/3
  Constant/1 -> Mux/1
  Power/1 -> Mux/2
  Mux/1 -> Gain/1
  B864/1(v) -> Power/1
  B864/2(i) -> Power/2
  Selector3/1 -> Scope1/2
  Gain1/1 -> Selector7/1, Selector3/1, Selector2/1
  Selector2/1 -> Scope1/1
  Power1/2 -> Mux1/3
  Constant1/1 -> Mux1/1
  Power1/1 -> Mux1/2
  Mux1/1 -> Gain1/1
  B1/1(v) -> Power1/1
  B1/2(i) -> Power1/2
  Selector5/1 -> Scope2/2
  Gain2/1 -> Selector8/1, Selector5/1, Selector4/1
  Selector4/1 -> Scope2/1
  Power2/2 -> Mux2/3
  Constant2/1 -> Mux2/1
  Power2/1 -> Mux2/2
  Mux2/1 -> Gain2/1
  B2/1(v) -> Power2/1
  B2/2(i) -> Power2/2
  Selector7/1 -> Mux3/2
  Selector6/1 -> Mux3/1
  Selector8/1 -> Mux3/3
  Mux3/1 -> To File/1
  connections:
  Load B/LConn2 -- Ground4/LConn1
  Load B1/LConn2 -- Ground5/LConn1
  Load B2/LConn2 -- Ground6/LConn1
  B864/RConn1 -- Load B/LConn1
  A/RConn1 -- B864/LConn1
  B1/RConn1 -- Load B1/LConn1
  B/RConn1 -- B1/LConn1
  B2/RConn1 -- Load B2/LConn1
  C/RConn1 -- B2/LConn1

== system IEEE34_SPSload/SM_IEEE34/Spot 890 ==
  Load B : Subsystem  DialogController=POWERSYS.PowerSysDialog  mask(Single-Phase Dynamic Load){NominalVoltage=[ VxfmL 60 ], ActiveReactivePowers=[150*1000*loadcoeff 75*1000*loadcoeff], PositiveSequence=[1 0], ExternalControl=off, NpNq=[1 1], TimeConstants=[0  0  0  0], MinimumVoltage=0.7, LoadFlowParameters=[4,0,0,0,0]}
      mask prompts: NominalVoltage "Nominal voltage and frequency  [Vn(Vrms) fn(Hz)]:"; ActiveReactivePowers "Active and reactive power at initial voltage [Po(W) Qo(var)]:"; PositiveSequence "Initial voltage Vo [Mag(pu) Phase (deg.)]:"; ExternalControl "External control of PQ"; NpNq "Parameters [ np  nq ]:"; TimeConstants "Time constants [Tp1 Tp2 Tq1 Tq2]  (s):"; MinimumVoltage "Minimum voltage Vmin (pu):"; LoadFlowParameters "Load Flow parameters"
      mask help:
      | Implements a single-phase dynamic load. Active  power P and reactive
      | power Q absorbed by the load vary as function of voltage V  according to the
      | following equations:
      |
      |   If V>Vmin, P and Q vary as follows:
      |        P = Po * (V/Vo)^np * (1+Tp1.s)/(1+Tp2.s)
      |        Q = Qo * (V/Vo)^nq * (1+Tq1.s)/(1+Tq2.s)
      |   if V<Vmin
      |      Same equations with np=nq=2 (constant impedance load)
      mask init: same as IEEE34_SPSload/SM_IEEE34/DL836-1/Load B
      mask Help: helpview(psbhelp)
      mask Callback ExternalControl: powericon('ThreePhaseDynamicLoadCback',gcb);
      mask Display:
      | plot(-45,-45,45,45,[0,9,18,24,29,30,29,24,18,9,0,-9,-18,-24,-29,-30,-29,-24,-18,-9,0]*.9,[30,29,24,18,9,0,-9,-18,-24,-29,-30,-29,-24,-18,-9,0,9,18,24,29,30]*.9)
      | plot([0,0,10,0,-10,0]*1.1,[15,-5,-5,-15,-5,-5]*1.1)
  Load B1 : Subsystem  DialogController=POWERSYS.PowerSysDialog  mask(Single-Phase Dynamic Load){NominalVoltage=[ VxfmL 60 ], ActiveReactivePowers=[150*1000*loadcoeff 75*1000*loadcoeff], PositiveSequence=[1 0], ExternalControl=off, NpNq=[1 1], TimeConstants=[0  0  0  0], MinimumVoltage=0.7, LoadFlowParameters=[4,0,0,0,0]}
      mask prompts: NominalVoltage "Nominal voltage and frequency  [Vn(Vrms) fn(Hz)]:"; ActiveReactivePowers "Active and reactive power at initial voltage [Po(W) Qo(var)]:"; PositiveSequence "Initial voltage Vo [Mag(pu) Phase (deg.)]:"; ExternalControl "External control of PQ"; NpNq "Parameters [ np  nq ]:"; TimeConstants "Time constants [Tp1 Tp2 Tq1 Tq2]  (s):"; MinimumVoltage "Minimum voltage Vmin (pu):"; LoadFlowParameters "Load Flow parameters"
      mask help:
      | Implements a single-phase dynamic load. Active  power P and reactive
      | power Q absorbed by the load vary as function of voltage V  according to the
      | following equations:
      |
      |   If V>Vmin, P and Q vary as follows:
      |        P = Po * (V/Vo)^np * (1+Tp1.s)/(1+Tp2.s)
      |        Q = Qo * (V/Vo)^nq * (1+Tq1.s)/(1+Tq2.s)
      |   if V<Vmin
      |      Same equations with np=nq=2 (constant impedance load)
      mask init: same as IEEE34_SPSload/SM_IEEE34/DL836-1/Load B
      mask Help: helpview(psbhelp)
      mask Callback ExternalControl: powericon('ThreePhaseDynamicLoadCback',gcb);
      mask Display:
      | plot(-45,-45,45,45,[0,9,18,24,29,30,29,24,18,9,0,-9,-18,-24,-29,-30,-29,-24,-18,-9,0]*.9,[30,29,24,18,9,0,-9,-18,-24,-29,-30,-29,-24,-18,-9,0,9,18,24,29,30]*.9)
      | plot([0,0,10,0,-10,0]*1.1,[15,-5,-5,-15,-5,-5]*1.1)
  Load B2 : Subsystem  DialogController=POWERSYS.PowerSysDialog  mask(Single-Phase Dynamic Load){NominalVoltage=[ VxfmL 60 ], ActiveReactivePowers=[150*1000*loadcoeff 75*1000*loadcoeff], PositiveSequence=[1 0], ExternalControl=off, NpNq=[1 1], TimeConstants=[0  0  0  0], MinimumVoltage=0.7, LoadFlowParameters=[4,0,0,0,0]}
      mask prompts: NominalVoltage "Nominal voltage and frequency  [Vn(Vrms) fn(Hz)]:"; ActiveReactivePowers "Active and reactive power at initial voltage [Po(W) Qo(var)]:"; PositiveSequence "Initial voltage Vo [Mag(pu) Phase (deg.)]:"; ExternalControl "External control of PQ"; NpNq "Parameters [ np  nq ]:"; TimeConstants "Time constants [Tp1 Tp2 Tq1 Tq2]  (s):"; MinimumVoltage "Minimum voltage Vmin (pu):"; LoadFlowParameters "Load Flow parameters"
      mask help:
      | Implements a single-phase dynamic load. Active  power P and reactive
      | power Q absorbed by the load vary as function of voltage V  according to the
      | following equations:
      |
      |   If V>Vmin, P and Q vary as follows:
      |        P = Po * (V/Vo)^np * (1+Tp1.s)/(1+Tp2.s)
      |        Q = Qo * (V/Vo)^nq * (1+Tq1.s)/(1+Tq2.s)
      |   if V<Vmin
      |      Same equations with np=nq=2 (constant impedance load)
      mask init: same as IEEE34_SPSload/SM_IEEE34/DL836-1/Load B
      mask Help: helpview(psbhelp)
      mask Callback ExternalControl: powericon('ThreePhaseDynamicLoadCback',gcb);
      mask Display:
      | plot(-45,-45,45,45,[0,9,18,24,29,30,29,24,18,9,0,-9,-18,-24,-29,-30,-29,-24,-18,-9,0]*.9,[30,29,24,18,9,0,-9,-18,-24,-29,-30,-29,-24,-18,-9,0,9,18,24,29,30]*.9)
      | plot([0,0,10,0,-10,0]*1.1,[15,-5,-5,-15,-5,-5]*1.1)
  Terminator : Terminator
  Terminator1 : Terminator
  Terminator2 : Terminator
  A : PMIOPort  Side=Right
  B : PMIOPort  Port=2  Side=Right
  C : PMIOPort  Port=3  Side=Right
  wires:
  Load B/1(m) -> Terminator/1
  Load B1/1(m) -> Terminator1/1
  Load B2/1(m) -> Terminator2/1
  connections:
  A/RConn1 -- Load B2/LConn2 -- Load B/LConn1
  B/RConn1 -- Load B/LConn2 -- Load B1/LConn1
  C/RConn1 -- Load B1/LConn2 -- Load B2/LConn1

== system IEEE34_SPSload/SM_IEEE34/DL836-1/Load B ==
  Controlled Current Source : spsControlledCurrentSourceLib/Controlled Current Source  Initialize=on  Source_Type=AC  Amplitude=0  Phase=0  Frequency=0  Measurements=None
  Gain : Gain  Gain=-1
  Measurement list : Subsystem
  PQ : Ground
  Series RLC Branch : spsSeriesRLCBranchLib/Series RLC Branch  LConnTagsString=__new0  RConnTagsString=__new0  BranchType=R  Resistance=1e8  Inductance=1e-3  SetiL0=off  InitialCurrent=0  Capacitance=1e-6  Setx0=off  InitialVoltage=0  Measurements=None
  Voltage Measurement1 : spsVoltageMeasurementLib/Voltage Measurement  PhasorSimulation=off  OutputType=Complex  PSBequivalent=0
  model : Subsystem
  a : PMIOPort  Tag=PMCPort  Side=Left
  b : PMIOPort  Tag=PMCPort  Port=2  Side=Left
  m : Outport  InitialOutput=[0,0,0]  VectorParamsAs1DForOutWhenUnconnected=off
  wires:
  Gain/1 -> Controlled Current Source/1
  Measurement list/1(Out1) -> m/1
  model/1(i) -> Gain/1
  Voltage Measurement1/1 -> model/1(v)
  PQ/1 -> model/2(PQ)
  model/2(m) -> Measurement list/1(In1)
  connections:
  Controlled Current Source/LConn1 -- b/RConn1 -- Series RLC Branch/RConn1 -- Voltage Measurement1/LConn2
  Controlled Current Source/RConn1 -- a/RConn1 -- Series RLC Branch/LConn1 -- Voltage Measurement1/LConn1

== system IEEE34_SPSload/SM_IEEE34/DL836-1/Load B1 ==
  Controlled Current Source : spsControlledCurrentSourceLib/Controlled Current Source  Initialize=on  Source_Type=AC  Amplitude=0  Phase=0  Frequency=0  Measurements=None
  Gain : Gain  Gain=-1
  Measurement list : Subsystem
  PQ : Ground
  Series RLC Branch : spsSeriesRLCBranchLib/Series RLC Branch  LConnTagsString=__new0  RConnTagsString=__new0  BranchType=R  Resistance=1e8  Inductance=1e-3  SetiL0=off  InitialCurrent=0  Capacitance=1e-6  Setx0=off  InitialVoltage=0  Measurements=None
  Voltage Measurement1 : spsVoltageMeasurementLib/Voltage Measurement  PhasorSimulation=off  OutputType=Complex  PSBequivalent=0
  model : Subsystem
  a : PMIOPort  Tag=PMCPort  Side=Left
  b : PMIOPort  Tag=PMCPort  Port=2  Side=Left
  m : Outport  InitialOutput=[0,0,0]  VectorParamsAs1DForOutWhenUnconnected=off
  wires:
  Gain/1 -> Controlled Current Source/1
  Measurement list/1(Out1) -> m/1
  model/1(i) -> Gain/1
  Voltage Measurement1/1 -> model/1(v)
  PQ/1 -> model/2(PQ)
  model/2(m) -> Measurement list/1(In1)
  connections:
  Controlled Current Source/LConn1 -- b/RConn1 -- Series RLC Branch/RConn1 -- Voltage Measurement1/LConn2
  Controlled Current Source/RConn1 -- a/RConn1 -- Series RLC Branch/LConn1 -- Voltage Measurement1/LConn1

== system IEEE34_SPSload/SM_IEEE34/DL836-1/Load B2 ==
  Controlled Current Source : spsControlledCurrentSourceLib/Controlled Current Source  Initialize=on  Source_Type=AC  Amplitude=0  Phase=0  Frequency=0  Measurements=None
  Gain : Gain  Gain=-1
  Measurement list : Subsystem
  PQ : Ground
  Series RLC Branch : spsSeriesRLCBranchLib/Series RLC Branch  LConnTagsString=__new0  RConnTagsString=__new0  BranchType=R  Resistance=1e8  Inductance=1e-3  SetiL0=off  InitialCurrent=0  Capacitance=1e-6  Setx0=off  InitialVoltage=0  Measurements=None
  Voltage Measurement1 : spsVoltageMeasurementLib/Voltage Measurement  PhasorSimulation=off  OutputType=Complex  PSBequivalent=0
  model : Subsystem
  a : PMIOPort  Tag=PMCPort  Side=Left
  b : PMIOPort  Tag=PMCPort  Port=2  Side=Left
  m : Outport  InitialOutput=[0,0,0]  VectorParamsAs1DForOutWhenUnconnected=off
  wires:
  model/2(m) -> Measurement list/1(In1)
  PQ/1 -> model/2(PQ)
  Voltage Measurement1/1 -> model/1(v)
  model/1(i) -> Gain/1
  Measurement list/1(Out1) -> m/1
  Gain/1 -> Controlled Current Source/1
  connections:
  Voltage Measurement1/LConn1 -- Series RLC Branch/LConn1 -- a/RConn1 -- Controlled Current Source/RConn1
  Voltage Measurement1/LConn2 -- Series RLC Branch/RConn1 -- b/RConn1 -- Controlled Current Source/LConn1

== system IEEE34_SPSload/SM_IEEE34/DL836-840/Load B ==
  Controlled Current Source : spsControlledCurrentSourceLib/Controlled Current Source  Initialize=on  Source_Type=AC  Amplitude=0  Phase=0  Frequency=0  Measurements=None
  Gain : Gain  Gain=-1
  Measurement list : Subsystem
  PQ : Ground
  Series RLC Branch : spsSeriesRLCBranchLib/Series RLC Branch  LConnTagsString=__new0  RConnTagsString=__new0  BranchType=R  Resistance=1e8  Inductance=1e-3  SetiL0=off  InitialCurrent=0  Capacitance=1e-6  Setx0=off  InitialVoltage=0  Measurements=None
  Voltage Measurement1 : spsVoltageMeasurementLib/Voltage Measurement  PhasorSimulation=off  OutputType=Complex  PSBequivalent=0
  model : Subsystem
  a : PMIOPort  Tag=PMCPort  Side=Left
  b : PMIOPort  Tag=PMCPort  Port=2  Side=Left
  m : Outport  InitialOutput=[0,0,0]  VectorParamsAs1DForOutWhenUnconnected=off
  wires:
  model/2(m) -> Measurement list/1(In1)
  PQ/1 -> model/2(PQ)
  Voltage Measurement1/1 -> model/1(v)
  model/1(i) -> Gain/1
  Measurement list/1(Out1) -> m/1
  Gain/1 -> Controlled Current Source/1
  connections:
  Voltage Measurement1/LConn1 -- Series RLC Branch/LConn1 -- a/RConn1 -- Controlled Current Source/RConn1
  Voltage Measurement1/LConn2 -- Series RLC Branch/RConn1 -- b/RConn1 -- Controlled Current Source/LConn1

== system IEEE34_SPSload/SM_IEEE34/DL836-840/Load B1 ==
  Controlled Current Source : spsControlledCurrentSourceLib/Controlled Current Source  Initialize=on  Source_Type=AC  Amplitude=0  Phase=0  Frequency=0  Measurements=None
  Gain : Gain  Gain=-1
  Measurement list : Subsystem
  PQ : Ground
  Series RLC Branch : spsSeriesRLCBranchLib/Series RLC Branch  LConnTagsString=__new0  RConnTagsString=__new0  BranchType=R  Resistance=1e8  Inductance=1e-3  SetiL0=off  InitialCurrent=0  Capacitance=1e-6  Setx0=off  InitialVoltage=0  Measurements=None
  Voltage Measurement1 : spsVoltageMeasurementLib/Voltage Measurement  PhasorSimulation=off  OutputType=Complex  PSBequivalent=0
  model : Subsystem
  a : PMIOPort  Tag=PMCPort  Side=Left
  b : PMIOPort  Tag=PMCPort  Port=2  Side=Left
  m : Outport  InitialOutput=[0,0,0]  VectorParamsAs1DForOutWhenUnconnected=off
  wires:
  model/2(m) -> Measurement list/1(In1)
  PQ/1 -> model/2(PQ)
  Voltage Measurement1/1 -> model/1(v)
  model/1(i) -> Gain/1
  Measurement list/1(Out1) -> m/1
  Gain/1 -> Controlled Current Source/1
  connections:
  Voltage Measurement1/LConn1 -- Series RLC Branch/LConn1 -- a/RConn1 -- Controlled Current Source/RConn1
  Voltage Measurement1/LConn2 -- Series RLC Branch/RConn1 -- b/RConn1 -- Controlled Current Source/LConn1

== system IEEE34_SPSload/SM_IEEE34/DL836-840/Load B2 ==
  Controlled Current Source : spsControlledCurrentSourceLib/Controlled Current Source  Initialize=on  Source_Type=AC  Amplitude=0  Phase=0  Frequency=0  Measurements=None
  Gain : Gain  Gain=-1
  Measurement list : Subsystem
  PQ : Ground
  Series RLC Branch : spsSeriesRLCBranchLib/Series RLC Branch  LConnTagsString=__new0  RConnTagsString=__new0  BranchType=R  Resistance=1e8  Inductance=1e-3  SetiL0=off  InitialCurrent=0  Capacitance=1e-6  Setx0=off  InitialVoltage=0  Measurements=None
  Voltage Measurement1 : spsVoltageMeasurementLib/Voltage Measurement  PhasorSimulation=off  OutputType=Complex  PSBequivalent=0
  model : Subsystem
  a : PMIOPort  Tag=PMCPort  Side=Left
  b : PMIOPort  Tag=PMCPort  Port=2  Side=Left
  m : Outport  InitialOutput=[0,0,0]  VectorParamsAs1DForOutWhenUnconnected=off
  wires:
  Gain/1 -> Controlled Current Source/1
  Measurement list/1(Out1) -> m/1
  model/1(i) -> Gain/1
  Voltage Measurement1/1 -> model/1(v)
  PQ/1 -> model/2(PQ)
  model/2(m) -> Measurement list/1(In1)
  connections:
  Controlled Current Source/LConn1 -- b/RConn1 -- Series RLC Branch/RConn1 -- Voltage Measurement1/LConn2
  Controlled Current Source/RConn1 -- a/RConn1 -- Series RLC Branch/LConn1 -- Voltage Measurement1/LConn1

== system IEEE34_SPSload/SM_IEEE34/DL862-1/Load B ==
  Controlled Current Source : spsControlledCurrentSourceLib/Controlled Current Source  Initialize=on  Source_Type=AC  Amplitude=0  Phase=0  Frequency=0  Measurements=None
  Gain : Gain  Gain=-1
  Measurement list : Subsystem
  PQ : Ground
  Series RLC Branch : spsSeriesRLCBranchLib/Series RLC Branch  LConnTagsString=__new0  RConnTagsString=__new0  BranchType=R  Resistance=1e8  Inductance=1e-3  SetiL0=off  InitialCurrent=0  Capacitance=1e-6  Setx0=off  InitialVoltage=0  Measurements=None
  Voltage Measurement1 : spsVoltageMeasurementLib/Voltage Measurement  PhasorSimulation=off  OutputType=Complex  PSBequivalent=0
  model : Subsystem
  a : PMIOPort  Tag=PMCPort  Side=Left
  b : PMIOPort  Tag=PMCPort  Port=2  Side=Left
  m : Outport  InitialOutput=[0,0,0]  VectorParamsAs1DForOutWhenUnconnected=off
  wires:
  Gain/1 -> Controlled Current Source/1
  Measurement list/1(Out1) -> m/1
  model/1(i) -> Gain/1
  Voltage Measurement1/1 -> model/1(v)
  PQ/1 -> model/2(PQ)
  model/2(m) -> Measurement list/1(In1)
  connections:
  Controlled Current Source/LConn1 -- b/RConn1 -- Series RLC Branch/RConn1 -- Voltage Measurement1/LConn2
  Controlled Current Source/RConn1 -- a/RConn1 -- Series RLC Branch/LConn1 -- Voltage Measurement1/LConn1

== system IEEE34_SPSload/SM_IEEE34/DL862-838/Load B ==
  Controlled Current Source : spsControlledCurrentSourceLib/Controlled Current Source  Initialize=on  Source_Type=AC  Amplitude=0  Phase=0  Frequency=0  Measurements=None
  Gain : Gain  Gain=-1
  Measurement list : Subsystem
  PQ : Ground
  Series RLC Branch : spsSeriesRLCBranchLib/Series RLC Branch  LConnTagsString=__new0  RConnTagsString=__new0  BranchType=R  Resistance=1e8  Inductance=1e-3  SetiL0=off  InitialCurrent=0  Capacitance=1e-6  Setx0=off  InitialVoltage=0  Measurements=None
  Voltage Measurement1 : spsVoltageMeasurementLib/Voltage Measurement  PhasorSimulation=off  OutputType=Complex  PSBequivalent=0
  model : Subsystem
  a : PMIOPort  Tag=PMCPort  Side=Left
  b : PMIOPort  Tag=PMCPort  Port=2  Side=Left
  m : Outport  InitialOutput=[0,0,0]  VectorParamsAs1DForOutWhenUnconnected=off
  wires:
  model/2(m) -> Measurement list/1(In1)
  PQ/1 -> model/2(PQ)
  Voltage Measurement1/1 -> model/1(v)
  model/1(i) -> Gain/1
  Measurement list/1(Out1) -> m/1
  Gain/1 -> Controlled Current Source/1
  connections:
  Voltage Measurement1/LConn1 -- Series RLC Branch/LConn1 -- a/RConn1 -- Controlled Current Source/RConn1
  Voltage Measurement1/LConn2 -- Series RLC Branch/RConn1 -- b/RConn1 -- Controlled Current Source/LConn1
